simulink model "bidirectional speed control using H-bridge"  (R2021a)
settings: Solver=VariableStepAuto  StartTime=0.0  StopTime=10.0  RelTol=1e-3
libraries: fl_lib x12, nesl_utility x6, spsMeanLib x1, spsPWMGeneratorDCDCLib x1
settings Model: Creator=hritw  LastModifiedBy=hritw

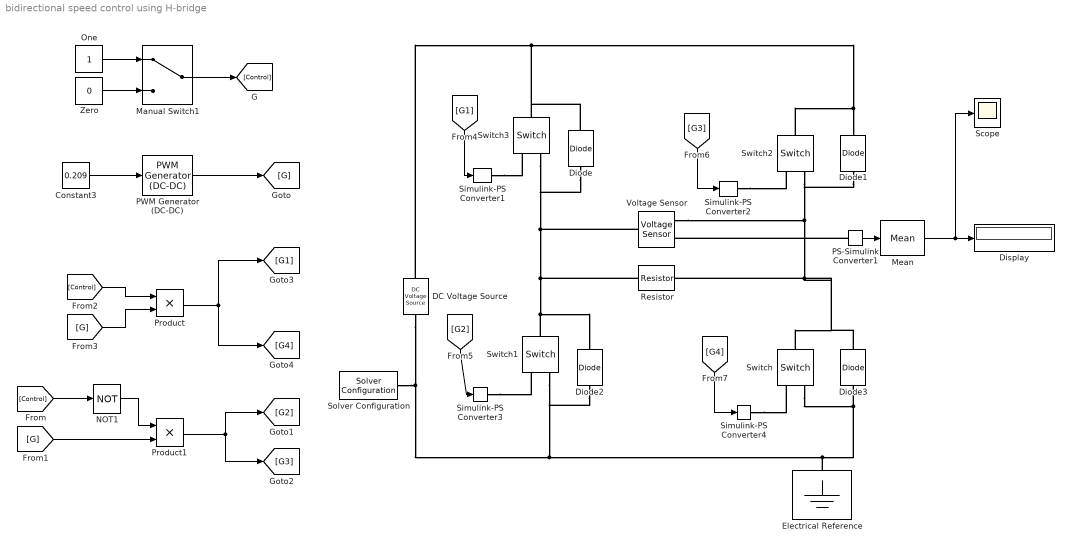
== system bidirectional speed control using H-bridge ==
  Constant3 : Constant  Value=0.209
  DC Voltage Source : fl_lib/Electrical/Electrical Sources/DC Voltage Source  v0=10 V
  Diode{,1..3} (4 alike) : fl_lib/Electrical/Electrical Elements/Diode  Vf=0.6 V  Ron=0.3 Ohm  Goff=1e-8 1/Ohm  i_specify=off  i_priority=None  i=0 A  i_nominal_specify=off  i_nominal_unit=A  i_nominal_value=1  v_specify=off  v_priority=None  v=0 V  v_nominal_specify=off  v_nominal_unit=V  v_nominal_value=1
  Display : Display
  Electrical Reference : fl_lib/Electrical/Electrical Elements/Electrical Reference
  Manual Switch1 : ManualSwitch
  Mean : spsMeanLib/Mean  Freq=60  Vinit=0  Ts=0
  NOT1 : Logic  Operator=NOT  IconShape=distinctive  AllPortsSameDT=off  OutDataTypeStr=boolean
  One : Constant  OutDataTypeStr=Inherit: Inherit via back propagation
  PS-Simulink Converter1 : nesl_utility/PS-Simulink Converter  PhysicalDomain=network_engine_domain  SubClassName=ps_output  LeftPortType=input  RightPortType=output  PseudoPeriodic=off  Frequencies=[]  Unit=inherit  AffineConversion=off
      settings: SourceProductBaseCode=PW,SS
  PWM Generator (DC-DC) : spsPWMGeneratorDCDCLib/PWM Generator (DC-DC)  Fsw=1000  Ts=0
  Product : Product
  Product1 : Product
  Resistor : fl_lib/Electrical/Electrical Elements/Resistor  R=1 kOhm  i_specify=off  i_priority=None  i=0 A  i_nominal_specify=off  i_nominal_unit=A  i_nominal_value=1  v_specify=off  v_priority=None  v=0 V  v_nominal_specify=off  v_nominal_unit=V  v_nominal_value=1
  Scope : Scope
  Simulink-PS Converter{1..4} (4 alike) : nesl_utility/Simulink-PS Converter  PhysicalDomain=network_engine_domain  SubClassName=ps_input  LeftPortType=input  RightPortType=output  PseudoPeriodic=off  Frequencies=[]  NoiseDistribution=none  NoiseParameters=[]  Unit=1  AffineConversion=off  FilteringAndDerivatives=provide  SimscapeFilterOrder=1  InputFilterTimeConstant=0.001  UdotUserProvided=0
      settings: SourceProductBaseCode=PW,SS
  Solver Configuration : nesl_utility/Solver Configuration  PhysicalDomain=network_engine_domain  SubClassName=solver  LeftPortType=input  RightPortType=generic  Tones=[]  Harmonics=[]  SimulateNoise=off  Profile=off  UseLocalSampling=off  EnableSwitchedLinearOptims=on  FrequencyDomain=off  UseCCode=off  RelTol=0.001  AbsTol=1e-06  MinStep=1e-09  ToWorkspace=off  RevertToSquareIcSolve=off  NumHomotopyIterations=100  PhasorMode=off  PhasorModeNumHarmonics=1  DoDC=off  ResidualTolerance=1e-09  UseLocalSolver=off  LocalSolverChoice=NE_BACKWARD_EULER_ADVANCER  LocalSolverSampleTime=0.001  DoFixedCost=off  MaxNonlinIter=3  MaxModeIter=2  ComputeImpulses=off  ImpulseIterations=2  LinearAlgebra=auto  EquationFormulation=NE_TIME_EF  DelaysMemoryBudget=1024  AutomaticFiltering=on  FilteringTimeConstant=0.001  PartitionStorageMethod=AS_NEEDED  PartitionMemoryBudget=1024  PartitionMethod=ROBUST
      settings: SourceProductBaseCode=PW,SS
  Switch{,1..3} (4 alike) : fl_lib/Electrical/Electrical Elements/Switch  R_closed=0.01 Ohm  G_open=1e-8 1/Ohm  Threshold=0.5  i_specify=off  i_priority=None  i=0 A  i_nominal_specify=off  i_nominal_unit=A  i_nominal_value=1  v_specify=off  v_priority=None  v=0 V  v_nominal_specify=off  v_nominal_unit=V  v_nominal_value=1
  Voltage Sensor : fl_lib/Electrical/Electrical Sensors/Voltage Sensor
  Zero : Constant  Value=0  OutDataTypeStr=Inherit: Inherit via back propagation
  wires:
  Manual Switch1/1 -> [Control]
  Product/1 -> [G4], [G1]
  Product1/1 -> [G3], [G2]
  One/1 -> Manual Switch1/1
  Zero/1 -> Manual Switch1/2
  [Control] -> NOT1/1
  PWM Generator (DC-DC)/1 -> [G]
  [G] -> Product/2
  [G1] -> Simulink-PS Converter1/1
  [G2] -> Simulink-PS Converter3/1
  [G3] -> Simulink-PS Converter2/1
  [G4] -> Simulink-PS Converter4/1
  [Control] -> Product/1
  [G] -> Product1/2
  NOT1/1 -> Product1/1
  Constant3/1 -> PWM Generator (DC-DC)/1
  PS-Simulink Converter1/1 -> Mean/1
  Mean/1 -> Scope/1, Display/1
  connections:
  Simulink-PS Converter3/RConn1 -- Switch1/RConn1
  DC Voltage Source/LConn1 -- Diode/RConn1 -- Switch3/LConn1 -- Switch2/LConn1 -- Diode1/RConn1
  Voltage Sensor/RConn2 -- Diode1/LConn1 -- Switch2/RConn2 -- Diode3/RConn1 -- Switch/LConn1 -- Resistor/RConn1
  PS-Simulink Converter1/LConn1 -- Voltage Sensor/RConn1
  DC Voltage Source/RConn1 -- Diode2/LConn1 -- Switch1/RConn2 -- Electrical Reference/LConn1 -- Switch/RConn2 -- Diode3/LConn1 -- Solver Configuration/RConn1
  Simulink-PS Converter2/RConn1 -- Switch2/RConn1
  Simulink-PS Converter4/RConn1 -- Switch/RConn1
  Switch1/LConn1 -- Resistor/LConn1 -- Voltage Sensor/LConn1 -- Diode/LConn1 -- Switch3/RConn2 -- Diode2/RConn1
  Simulink-PS Converter1/RConn1 -- Switch3/RConn1
